simulink model "lidar_tester3"  (Simulink 7.3)
settings: Solver=FixedStepDiscrete  StartTime=0.0  StopTime=inf  RelTol=1e-3
settings Model: Creator=wildcat  LastModifiedBy=wildcat
settings DebuggingCC: FcnCallInpInsideContextMsg=Enable All  StrictBusMsg=ErrorLevel1
settings SFSimCC: SimUserLibraries=phidget21
settings RTWCC: SystemTargetFile=rlnx.tlc  GenCodeOnly=on  TemplateMakefile=rlnx_ubuntu.tmf  Description=Linux Real-Time Target  ProcessScript=rlnx_make_rtw_hook
settings RTWCC: CustomInclude=|
  | /home/wesley/Desktop/libphidget-2.1.8.20140319/
  | /home/wesley/Desktop/FAUTest/TestWithNoVideo/
settings CodeAppCC: GenerateComments=off  SimulinkBlockComments=off
settings STFCustomTargetCC: ModelReferenceCompliant=off  MatFileLogging=on  SystemTargetFile=rlnx.tlc
settings GRTTargetCC: ModelReferenceCompliant=off  ParMdlRefBuildCompliant=off  CompOptLevelCompliant=off
settings CustomProperty: DataType=string  Value=-lm -ldl -lc_urg -lc_urg_connection -lc_urg_system -lphidget21
settings EnumStrPairs: String=PC

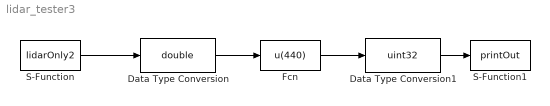
== system lidar_tester3 ==
  Data Type Conversion : DataTypeConversion  OutDataTypeMode=double  OutDataType=fixdt(1, 16)  OutScaling=2^0  OutDataTypeStr=double
  Data Type Conversion1 : DataTypeConversion  OutDataTypeMode=uint32  OutDataType=fixdt(1, 16)  OutScaling=2^0  OutDataTypeStr=uint32
  Fcn : Fcn  Expr=u(440)
  S-Function : S-Function  FunctionName=lidarOnly2  EnableBusSupport=off
  S-Function1 : S-Function  FunctionName=printOut  EnableBusSupport=off
  wires:
  Data Type Conversion1/1 -> S-Function1/1
  Data Type Conversion/1 -> Fcn/1
  Fcn/1 -> Data Type Conversion1/1
  S-Function/1 -> Data Type Conversion/1
